simulink model "irep_force_control_m15"  (R2015a)
settings: Solver=ode3  StartTime=0.0  StopTime=inf  FixedStep=dt  RelTol=1e-3
InitFcn:
  | IREP_DEPENDENCY
  | init_omni
  | init_filters
  | init_invivo
  | init_telemanipulation
  | init_parker_xyz
  | init_magnetic_tracker
  | init_loadcell
  | init_scopes
  | init_homing
  | init_force_control
  | init_xpc_invivo_simu
undefined symbols (not defined in the file): ang_vel_scale, B_simu, beta, camera_home_voltage, counter_offset, dt, dt_trakstar, E_Y, encoder_counts, epsilon_robust_inverse, FS_LUT_TAU, FS_LUT_WE, gear_ratio, HomingFineEps, HomingRoughEps, HomingRoughVelocity, I1_primary, I1_secondary, I2_primary, I2_secondary, irep_parameters_left, irep_parameters_right, joystick_filter_coeffs, K_d, K_i, K_naive_inv, K_p, k_right, L1l, L1r, L2l, L2r, L_zeus, left_arm_home_voltage, left_x0_parallelogram, LeftArmHomingDirectionVector, LeftArmHomingIntGain, lin_vel_scale, LOADCELL_BIAS, LOADCELL_GAIN, max_conf_space_speed, N_joystick, N_pots, N_trakstar, OmegaMax, OmegaMin, orientation_epsilon, position_epsilon, pots_filter_coeffs, q_eps_backlash, quadrature_mode, r, right_arm_home_voltage, RightArmHomingDirectionVector, RightArmHomingIntGain, screw_pitch, statics_param, tau_compression_bias, tau_compression_gains, tau_neutral_deadband ... (+16)
libraries: slrtlib x39, simulink x23, xpcobsoletelib x23, xpcconteclib x23, xpcrtudplib x12, xpcmeasurementcomputinglib x6, dspswit3 x2, dspsigops x1
(part 5 of 7)

== system irep_force_control_m15/Trajectory Planner/Right Arm/High Level/Actuation Compensation/Grad U2 ==
  conf space : Inport
  q : Inport  Port=2
  Compute grad U : MATLAB Function  TreatAsAtomicUnit=on
  Constant : Constant  Value=L2r  SampleTime=dt
  E_Y : Constant  Value=E_Y  SampleTime=dt
  Ip : Constant  Value=I2_primary  SampleTime=dt
  Is : Constant  Value=I2_secondary  SampleTime=dt
  beta : Constant  Value=beta  SampleTime=dt
  r : Constant  Value=r  SampleTime=dt
  theta_0 : Constant  Value=theta0  SampleTime=dt
  grad_U : Outport
  wires:
  Is/1 -> Compute grad U/7(Is)
  q/1 -> Compute grad U/2(q)
  conf space/1 -> Compute grad U/1(conf_space)
  Compute grad U/1(grad_U) -> grad_U/1
  E_Y/1 -> Compute grad U/5(E_Y)
  Ip/1 -> Compute grad U/6(Ip)
  r/1 -> Compute grad U/4(r)
  theta_0/1 -> Compute grad U/8(theta_0)
  beta/1 -> Compute grad U/9(beta)
  Constant/1 -> Compute grad U/3(L_p)

== system irep_force_control_m15/Trajectory Planner/Right Arm/High Level/Actuation Compensation/Parallelogram Backlash Compensatior ==
  q des : Inport
  Backlash Compensator : MATLAB Function  TreatAsAtomicUnit=on
  Bus Selector : BusSelector  OutputSignals=q2;q3
  Discrete Derivative : simulink/Discrete/Discrete Derivative  gainval=1.0  ICPrevScaledInput=0.0  InputProcessing=Inherited  OutMin=[]  OutMax=[]  OutDataType=fixdt(1, 16)  OutScaling=2^-10  DoSatur=off
  comp close : Constant  Value=0
  comp close1 : Constant  Value=0.6
  comp open : Constant  Value=0
  comp open1 : Constant  Value=-1.2
  epsilon : Outport
  wires:
  q des/1 -> Bus Selector/1
  Bus Selector/1 -> Discrete Derivative/1, Backlash Compensator/1(q_curr)  "<q2;q3>"
  Discrete Derivative/1 -> Backlash Compensator/2(q_dot_curr)  "q dot curr"
  Backlash Compensator/1(epsilon) -> epsilon/1
  comp open/1 -> Backlash Compensator/3(q1_comp_open)
  comp close/1 -> Backlash Compensator/4(q1_comp_close)
  comp open1/1 -> Backlash Compensator/5(q2_comp_open)
  comp close1/1 -> Backlash Compensator/6(q2_comp_close)

== system irep_force_control_m15/Trajectory Planner/Right Arm/High Level/Actuation Compensation/get q_dot sign ==
  conf_space_dot : Inport
  conf_space : Inport  Port=2
  Dead Zone : DeadZone  LowerValue=-1e-3  UpperValue=1e-3  SaturateOnIntegerOverflow=on
  Unit Delay : UnitDelay  SampleTime=-1
  compute q_dot : MATLAB Function  TreatAsAtomicUnit=on
  hold q dot : MATLAB Function  TreatAsAtomicUnit=on
  q_dot : Outport
  wires:
  conf_space_dot/1 -> compute q_dot/2(conf_space_dot)
  conf_space/1 -> compute q_dot/1(conf_space)
  hold q dot/1(q_dot_sign_out) -> q_dot/1, Unit Delay/1
  Unit Delay/1 -> hold q dot/2(q_dot_sign_prev)
  compute q_dot/1(q_dot) -> Dead Zone/1
  Dead Zone/1 -> hold q dot/1(q_dot_sign_in)

== system irep_force_control_m15/Trajectory Planner/Right Arm/High Level/Actuation Compensation/q_eps 5th order poly ==
  q_eps_ref : Inport
  enable : Inport  Port=2
  Constant : Constant  Value=q_eps_backlash
  Digital Clock : DigitalClock  SampleTime=dt
  Embedded MATLAB Function : MATLAB Function  TreatAsAtomicUnit=on
  Terminator : Terminator
  Unit Delay : UnitDelay  SampleTime=dt
  Unit Delay1 : UnitDelay  SampleTime=dt
  Unit Delay2 : UnitDelay  InitialCondition=zeros(9,1)  SampleTime=dt
  tf : Constant  Value=5  SampleTime=dt
  q_eps_des : Outport
  wires:
  Embedded MATLAB Function/3(confn) -> Unit Delay/1
  Unit Delay/1 -> Embedded MATLAB Function/5(conf)
  Embedded MATLAB Function/4(t0n) -> Unit Delay1/1
  Embedded MATLAB Function/5(p0n) -> Unit Delay2/1
  Unit Delay2/1 -> Embedded MATLAB Function/7(p0)
  Unit Delay1/1 -> Embedded MATLAB Function/6(t0)
  Digital Clock/1 -> Embedded MATLAB Function/4(tc)
  q_eps_ref/1 -> Embedded MATLAB Function/1(p_des)
  Embedded MATLAB Function/1(p) -> q_eps_des/1
  tf/1 -> Embedded MATLAB Function/3(tf)
  enable/1 -> Embedded MATLAB Function/8(enable)
  Constant/1 -> Embedded MATLAB Function/2(p_curr)
  Embedded MATLAB Function/2(pdot) -> Terminator/1

== system irep_force_control_m15/Trajectory Planner/Right Arm/High Level/Configuration Space/Parallelogram ==
  Enable : EnablePort
  5th Order Polynomial : Subsystem
  b_des : Constant  Value=[x0_parallelogram z0_parallelogram]  SampleTime=dt
  b1 : Outport
  wires:
  b_des/1 -> 5th Order Polynomial/1(b des)
  5th Order Polynomial/1(b) -> b1/1

== system irep_force_control_m15/Trajectory Planner/Right Arm/High Level/Configuration Space/Stem ==
  Enable : EnablePort
  5th Order Polynomial : Subsystem
  Terminator : Terminator
  enable : Constant  Value=0  SampleTime=dt
  psi des : Constant  Value=[pi/2;0;pi/2;0;0]  SampleTime=dt
  psi0 : Constant  Value=[pi/2;0;pi/2;0;0]  SampleTime=dt
  psi dot : Outport  InitialOutput=zeros(5,1)
  wires:
  5th Order Polynomial/2(psi dot) -> psi dot/1
  psi des/1 -> 5th Order Polynomial/1(psi des)
  psi0/1 -> 5th Order Polynomial/2(psi0)
  enable/1 -> 5th Order Polynomial/3(enable)
  5th Order Polynomial/1(psi) -> Terminator/1

== system irep_force_control_m15/Trajectory Planner/Right Arm/High Level/Inverse Istantaneous Kinematics/Coordination Module ==
  b1 : Inport
  q par : Inport  Port=2
  5-Bar Inverse Kinematics : MATLAB Function  TreatAsAtomicUnit=on
  Add : Sum  Inputs=+-  SampleTime=dt
  Coordination Block : MATLAB Function  TreatAsAtomicUnit=on
  L0 : Constant  Value=L_zeus  SampleTime=dt
  b0 : Constant  Value=[x0_parallelogram z0_parallelogram]  SampleTime=dt
  q1 : Outport
  "q2, q3" : Outport  Port=2
  wires:
  Add/1 -> "q2, q3"/1
  q par/1 -> Coordination Block/2(q_par)
  b1/1 -> Coordination Block/1(b1)
  Coordination Block/1(q1) -> q1/1
  5-Bar Inverse Kinematics/1(q) -> Add/2
  L0/1 -> Coordination Block/3(L0)
  b0/1 -> 5-Bar Inverse Kinematics/1(b1)
  Coordination Block/2(q23) -> Add/1

== system irep_force_control_m15/Trajectory Planner/Right Arm/High Level/Inverse Istantaneous Kinematics/Jaw Open//Close Module ==
  sensors : Inport
  Enable : EnablePort
  Bus Selector : BusSelector  OutputSignals=MSG_Type,gripper
  Jaw Open/Close : MATLAB Function  TreatAsAtomicUnit=on
  MTM_GP_max : Constant  Value=1.05
  MTM_GP_min : Constant  Value=-0.48
  Unit Delay : UnitDelay  SampleTime=-1
  Unit Delay1 : UnitDelay  SampleTime=-1
  q9 : Outport
  wires:
  sensors/1 -> Bus Selector/1
  Jaw Open/Close/1(y) -> Unit Delay/1, Unit Delay1/1
  Bus Selector/2 -> Jaw Open/Close/2(u)  "<gripper>"
  MTM_GP_max/1 -> Jaw Open/Close/3(MTM_GP_max)
  MTM_GP_min/1 -> Jaw Open/Close/4(MTM_GP_min)
  Bus Selector/1 -> Jaw Open/Close/1(MSG_valid)  "<MSG_Type>"
  Unit Delay/1 -> Jaw Open/Close/5(q9_prev)
  Unit Delay1/1 -> q9/1

== system irep_force_control_m15/Trajectory Planner/Right Arm/High Level/Task Space/Compute Weigths ==
  sensors : Inport
  conf space : Inport  Port=2
  Bus Selector : BusSelector  OutputSignals=b1 curr,psi curr
  Bus Selector1 : BusSelector  OutputSignals=foot switches
  joint limits : Constant  Value=[x0_parallelogram x0_parallelogram_max z0_parallelogram z0_parallelogram_max theta_min1 theta_max theta_min2 theta_max wrist_min wrist_max]  SampleTime=dt
  select weights : MATLAB Function  TreatAsAtomicUnit=on
  w_min : Constant  Value=w_min  SampleTime=dt
  weights : Outport
  wires:
  joint limits/1 -> select weights/3(joint_limits)
  Bus Selector/1 -> select weights/1(b1)  "<b1 curr>"
  Bus Selector/2 -> select weights/2(psi)  "<psi curr>"
  conf space/1 -> Bus Selector/1
  select weights/1(W) -> weights/1
  w_min/1 -> select weights/4(w_min)
  sensors/1 -> Bus Selector1/1
  Bus Selector1/1 -> select weights/5(foot_switches)  "<foot switches>"

== system irep_force_control_m15/Trajectory Planner/Right Arm/High Level/Task Space/Desired Twist Module ==
  note: Desired Twist Module v 1.1 - © 2011 Andrea Bajo, Nabil Simaan
  current pose : Inport
  des pose : Inport  Port=2
  Bus Selector1 : BusSelector  OutputSignals=p in world,R in world
  Bus Selector2 : BusSelector  OutputSignals=position,R,MSG_Type
  Compute Twist : MATLAB Function  TreatAsAtomicUnit=on
  Omega Max : Constant  Value=OmegaMax  SampleTime=dt
  Omega Min : Constant  Value=OmegaMin  SampleTime=dt
  V Max : Constant  Value=Vmax  SampleTime=dt
  V Min : Constant  Value=Vmin  SampleTime=dt
  ang vel scale : Constant  Value=ang_vel_scale  SampleTime=dt
  lin vel scale : Constant  Value=lin_vel_scale  SampleTime=dt
  orientation epsilon : Constant  Value=orientation_epsilon  SampleTime=dt
  position epsilon : Constant  Value=position_epsilon  SampleTime=dt
  x des : Outport
  wires:
  Bus Selector1/1 -> Compute Twist/4(p_curr)  "<p in world>"
  Compute Twist/1(x_des) -> x des/1
  current pose/1 -> Bus Selector1/1
  Bus Selector1/2 -> Compute Twist/5(R_curr)  "<R in world>"
  Bus Selector2/1 -> Compute Twist/1(p_des)  "<position>"
  Bus Selector2/2 -> Compute Twist/2(R_des)  "<R>"
  des pose/1 -> Bus Selector2/1
  Bus Selector2/3 -> Compute Twist/3(MSG_Type)  "<MSG_Type>"
  V Max/1 -> Compute Twist/6(Vmax)
  Omega Max/1 -> Compute Twist/10(OmegaMax)
  V Min/1 -> Compute Twist/7(Vmin)
  Omega Min/1 -> Compute Twist/11(OmegaMin)
  position epsilon/1 -> Compute Twist/8(position_epsilon)
  orientation epsilon/1 -> Compute Twist/12(orientation_epsilon)
  lin vel scale/1 -> Compute Twist/9(lin_vel_scale)
  ang vel scale/1 -> Compute Twist/13(ang_vel_scale)

== system irep_force_control_m15/Trajectory Planner/Right Arm/High Level/Task Space/Direct Kinematics IREP ==
  "b1, psi" : Inport
  Bus Creator : BusCreator  Inputs=2
  Bus Selector : BusSelector  OutputSignals=Parker insertion stage,b1 curr,psi curr
  Direct Kinematic IREP : MATLAB Function  TreatAsAtomicUnit=on
  IREP parameters : Constant  Value=irep_parameters_right  SampleTime=dt
  Current Pose : Outport
  wires:
  "b1, psi"/1 -> Bus Selector/1
  Bus Selector/2 -> Direct Kinematic IREP/2(b1)  "<b1 curr>"
  Bus Selector/3 -> Direct Kinematic IREP/3(psi)  "<psi curr>"
  Direct Kinematic IREP/1(p) -> Bus Creator/1  "p in world"
  Direct Kinematic IREP/2(R) -> Bus Creator/2  "R in world"
  Bus Creator/1 -> Current Pose/1
  IREP parameters/1 -> Direct Kinematic IREP/4(parameters)
  Bus Selector/1 -> Direct Kinematic IREP/1(b0)  "<Parker insertion stage>"

== system irep_force_control_m15/Trajectory Planner/Right Arm/High Level/Task Space/Jxpsi Inverse IREP ==
  x des : Inport
  weights : Inport  Port=2
  "b1, psi" : Inport  Port=3
  Bus Selector : BusSelector  OutputSignals=Parker insertion stage,b1 curr,psi curr
  IREP parameters : Constant  Value=irep_parameters_right  SampleTime=dt
  Jxpsi Inverse IREP : MATLAB Function  TreatAsAtomicUnit=on
  epsilon : Constant  Value=epsilon_robust_inverse  SampleTime=dt
  max conf space speed : Constant  Value=max_conf_space_speed  SampleTime=dt
  conf dot des : Outport  PortDimensions=[8 1]
  wires:
  IREP parameters/1 -> Jxpsi Inverse IREP/5(parameters)
  x des/1 -> Jxpsi Inverse IREP/1(x_des)
  Bus Selector/3 -> Jxpsi Inverse IREP/4(psi)  "<psi curr>"
  Bus Selector/2 -> Jxpsi Inverse IREP/3(b1)  "<b1 curr>"
  "b1, psi"/1 -> Bus Selector/1
  Jxpsi Inverse IREP/1(conf_space_dot) -> conf dot des/1
  epsilon/1 -> Jxpsi Inverse IREP/7(epsilon_in)
  weights/1 -> Jxpsi Inverse IREP/6(weights)
  Bus Selector/1 -> Jxpsi Inverse IREP/2(b0)  "<Parker insertion stage>"
  max conf space speed/1 -> Jxpsi Inverse IREP/8(max_ang_speed)

== system irep_force_control_m15/Trajectory Planner/Right Arm/High Level/Task Space/Receive Desired Pose from MTM ==
  note: Telemanipulation Module v 1.0 - © COPYRIGHT 2010 Andrea Bajo, Nabil Simaan
  Master : Inport
  Bus Creator : BusCreator
  Bus Selector : BusSelector  OutputSignals=position,orientation (quat),MSG_Type,gripper
  Quaternion To Rotation : MATLAB Function  TreatAsAtomicUnit=on
  "pose, flags" : Outport
  wires:
  Bus Creator/1 -> "pose, flags"/1
  Master/1 -> Bus Selector/1
  Bus Selector/1 -> Bus Creator/1  "<position>"
  Quaternion To Rotation/1(R) -> Bus Creator/2
  Bus Selector/2 -> Quaternion To Rotation/1(quat)  "<orientation (quat)>"
  Bus Selector/3 -> Bus Creator/3  "<MSG_Type>"
  Bus Selector/4 -> Bus Creator/4  "<gripper>"

== system irep_force_control_m15/Trajectory Planner/Right Arm/High Level/Task Space/right task space scope ==
  des : Inport
  Bus Selector7 : BusSelector  OutputSignals=position,R,gripper,MSG_Type
  Gain : Gain
  Mux : Mux  Inputs=5
  R_to_axis_angle1 : MATLAB Function  TreatAsAtomicUnit=on
  right task space : slrtlib/Displays and Logging/Scope   scopeno=26  scopetype=Host  autostart=on  viewmode=Numerical  formatstr=scope_format_right_task_space_des  grid=on  ylimits=[0,0]  nosamples=10  noprepostsamples=0  interleave=1  triggermode=FreeRun  triggersignal=1  trigsignalfromport=off  triggerlevel=0.0  triggerslope=Either  triggerscope=1  triggersample=0  filename=weights1.dat  mode=Lazy  writesize=512  autorestart=off  dynamicfilemode=off  maxwritefilesize=512*1024^2
  wires:
  Mux/1 -> Gain/1
  des/1 -> Bus Selector7/1
  Bus Selector7/2 -> R_to_axis_angle1/1(R)  "<R>"
  Gain/1 -> right task space/1
  Bus Selector7/3 -> Mux/4  "<gripper>"
  R_to_axis_angle1/1(n_vec) -> Mux/2
  R_to_axis_angle1/2(theta) -> Mux/3
  Bus Selector7/1 -> Mux/1  "<position>"
  Bus Selector7/4 -> Mux/5  "<MSG_Type>"

== system irep_force_control_m15/Trajectory Planner/Right Arm/Low Level/Home Procedure/Fine Homing - Integral Control ==
  error : Inport
  Enable : EnablePort  StatesWhenEnabling=reset
  Discrete-Time Integrator : DiscreteIntegrator  SampleTime=dt  LimitOutput=on  UpperSaturationLimit=8  LowerSaturationLimit=-8
  Integral Gain : Gain  Gain=diag(RightArmHomingIntGain)  Multiplication=Matrix(K*u)  SampleTime=dt
  q_des_fine : Outport  InitialOutput=zeros(9,1)
  wires:
  error/1 -> Integral Gain/1
  Discrete-Time Integrator/1 -> q_des_fine/1
  Integral Gain/1 -> Discrete-Time Integrator/1

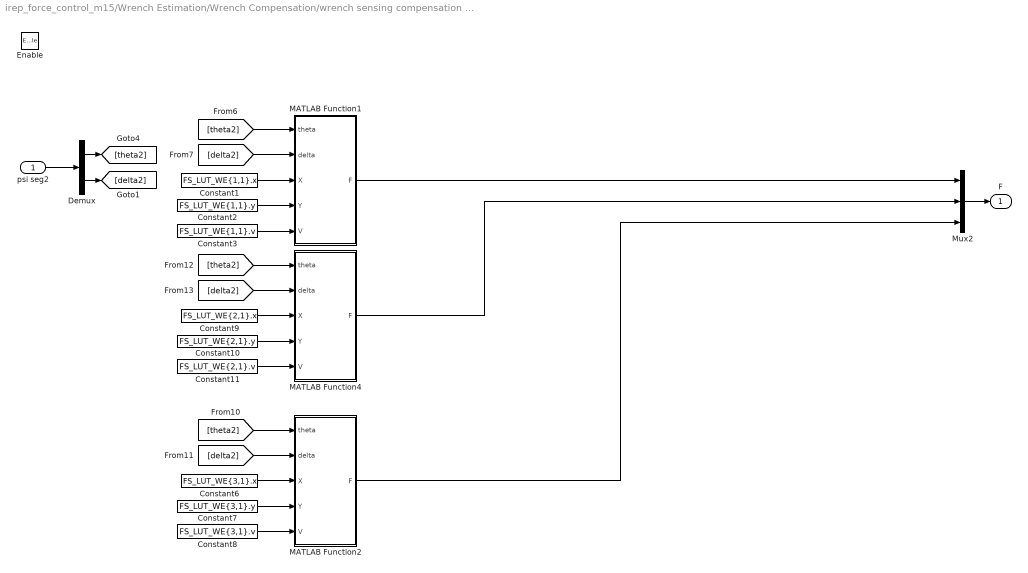
== system irep_force_control_m15/Wrench Estimation/Wrench Compensation/wrench sensing compensation LUT/wrench seg2 bias LUT/Interp2 Case A ==
  psi seg2 : Inport
  Enable : EnablePort
  Constant1 : Constant  Value=FS_LUT_WE{1,1}.x  VectorParams1D=off
  Constant10 : Constant  Value=FS_LUT_WE{2,1}.y  VectorParams1D=off
  Constant11 : Constant  Value=FS_LUT_WE{2,1}.v  VectorParams1D=off
  Constant2 : Constant  Value=FS_LUT_WE{1,1}.y  VectorParams1D=off
  Constant3 : Constant  Value=FS_LUT_WE{1,1}.v  VectorParams1D=off
  Constant6 : Constant  Value=FS_LUT_WE{3,1}.x  VectorParams1D=off
  Constant7 : Constant  Value=FS_LUT_WE{3,1}.y  VectorParams1D=off
  Constant8 : Constant  Value=FS_LUT_WE{3,1}.v  VectorParams1D=off
  Constant9 : Constant  Value=FS_LUT_WE{2,1}.x  VectorParams1D=off
  Demux : Demux  Outputs=2
  MATLAB Function1 : MATLAB Function  TreatAsAtomicUnit=on
  MATLAB Function2 : MATLAB Function  TreatAsAtomicUnit=on
  MATLAB Function4 : MATLAB Function  TreatAsAtomicUnit=on
  Mux2 : Mux  Inputs=3
  F : Outport
  wires:
  Constant3/1 -> MATLAB Function1/5(V)
  Constant2/1 -> MATLAB Function1/4(Y)
  Constant1/1 -> MATLAB Function1/3(X)
  [delta2] -> MATLAB Function1/2(delta)
  [theta2] -> MATLAB Function1/1(theta)
  Constant11/1 -> MATLAB Function4/5(V)
  Constant10/1 -> MATLAB Function4/4(Y)
  Constant9/1 -> MATLAB Function4/3(X)
  [delta2] -> MATLAB Function4/2(delta)
  [theta2] -> MATLAB Function4/1(theta)
  Constant8/1 -> MATLAB Function2/5(V)
  Constant7/1 -> MATLAB Function2/4(Y)
  Constant6/1 -> MATLAB Function2/3(X)
  [delta2] -> MATLAB Function2/2(delta)
  [theta2] -> MATLAB Function2/1(theta)
  MATLAB Function4/1(F) -> Mux2/2
  Mux2/1 -> F/1
  MATLAB Function1/1(F) -> Mux2/1
  MATLAB Function2/1(F) -> Mux2/3
  Demux/2 -> [delta2]
  Demux/1 -> [theta2]
  psi seg2/1 -> Demux/1

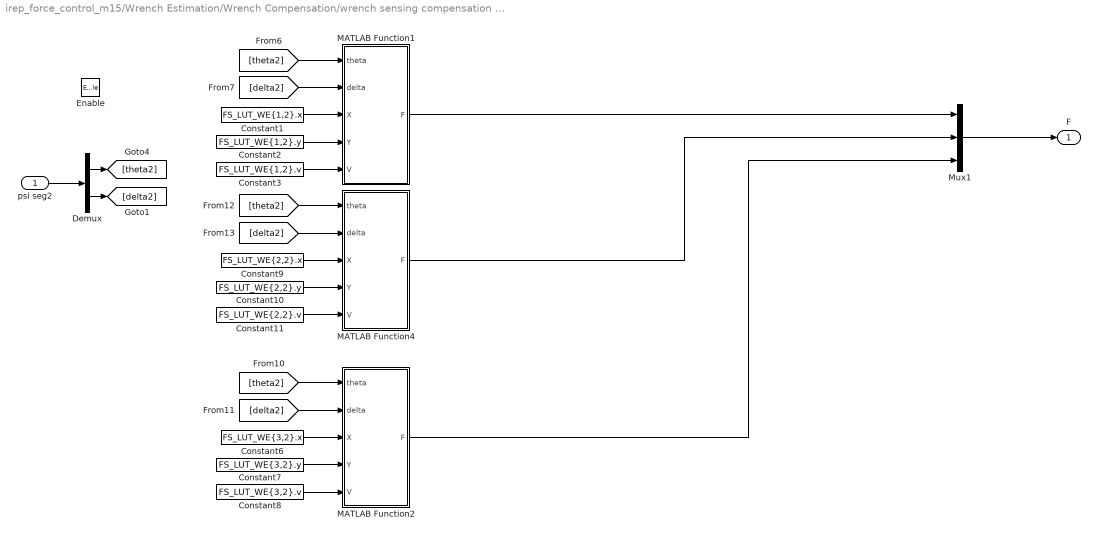
== system irep_force_control_m15/Wrench Estimation/Wrench Compensation/wrench sensing compensation LUT/wrench seg2 bias LUT/Interp2 Case B ==
  psi seg2 : Inport
  Enable : EnablePort
  Constant1 : Constant  Value=FS_LUT_WE{1,2}.x  VectorParams1D=off
  Constant10 : Constant  Value=FS_LUT_WE{2,2}.y  VectorParams1D=off
  Constant11 : Constant  Value=FS_LUT_WE{2,2}.v  VectorParams1D=off
  Constant2 : Constant  Value=FS_LUT_WE{1,2}.y  VectorParams1D=off
  Constant3 : Constant  Value=FS_LUT_WE{1,2}.v  VectorParams1D=off
  Constant6 : Constant  Value=FS_LUT_WE{3,2}.x  VectorParams1D=off
  Constant7 : Constant  Value=FS_LUT_WE{3,2}.y  VectorParams1D=off
  Constant8 : Constant  Value=FS_LUT_WE{3,2}.v  VectorParams1D=off
  Constant9 : Constant  Value=FS_LUT_WE{2,2}.x  VectorParams1D=off
  Demux : Demux  Outputs=2
  MATLAB Function1 : MATLAB Function  TreatAsAtomicUnit=on
  MATLAB Function2 : MATLAB Function  TreatAsAtomicUnit=on
  MATLAB Function4 : MATLAB Function  TreatAsAtomicUnit=on
  Mux1 : Mux  Inputs=3
  F : Outport
  wires:
  Constant3/1 -> MATLAB Function1/5(V)
  Constant2/1 -> MATLAB Function1/4(Y)
  Constant1/1 -> MATLAB Function1/3(X)
  [delta2] -> MATLAB Function1/2(delta)
  [theta2] -> MATLAB Function1/1(theta)
  Constant11/1 -> MATLAB Function4/5(V)
  Constant10/1 -> MATLAB Function4/4(Y)
  Constant9/1 -> MATLAB Function4/3(X)
  [delta2] -> MATLAB Function4/2(delta)
  [theta2] -> MATLAB Function4/1(theta)
  Constant8/1 -> MATLAB Function2/5(V)
  Constant7/1 -> MATLAB Function2/4(Y)
  Constant6/1 -> MATLAB Function2/3(X)
  [delta2] -> MATLAB Function2/2(delta)
  [theta2] -> MATLAB Function2/1(theta)
  MATLAB Function4/1(F) -> Mux1/2
  Mux1/1 -> F/1
  MATLAB Function1/1(F) -> Mux1/1
  MATLAB Function2/1(F) -> Mux1/3
  Demux/2 -> [delta2]
  Demux/1 -> [theta2]
  psi seg2/1 -> Demux/1

== system irep_force_control_m15/Wrench Estimation/Wrench Compensation/wrench sensing compensation LUT/wrench seg2 bias LUT/Interp2 Case C ==
  psi seg2 : Inport
  Enable : EnablePort
  Constant1 : Constant  Value=FS_LUT_WE{1,3}.x  VectorParams1D=off
  Constant10 : Constant  Value=FS_LUT_WE{2,3}.y  VectorParams1D=off
  Constant11 : Constant  Value=FS_LUT_WE{2,3}.v  VectorParams1D=off
  Constant2 : Constant  Value=FS_LUT_WE{1,3}.y  VectorParams1D=off
  Constant3 : Constant  Value=FS_LUT_WE{1,3}.v  VectorParams1D=off
  Constant6 : Constant  Value=FS_LUT_WE{3,3}.x  VectorParams1D=off
  Constant7 : Constant  Value=FS_LUT_WE{3,3}.y  VectorParams1D=off
  Constant8 : Constant  Value=FS_LUT_WE{3,3}.v  VectorParams1D=off
  Constant9 : Constant  Value=FS_LUT_WE{2,3}.x  VectorParams1D=off
  Demux : Demux  Outputs=2
  MATLAB Function1 : MATLAB Function  TreatAsAtomicUnit=on
  MATLAB Function2 : MATLAB Function  TreatAsAtomicUnit=on
  MATLAB Function4 : MATLAB Function  TreatAsAtomicUnit=on
  Mux2 : Mux  Inputs=3
  F1 : Outport
  wires:
  Constant3/1 -> MATLAB Function1/5(V)
  Constant2/1 -> MATLAB Function1/4(Y)
  Constant1/1 -> MATLAB Function1/3(X)
  [delta2] -> MATLAB Function1/2(delta)
  [theta2] -> MATLAB Function1/1(theta)
  Constant11/1 -> MATLAB Function4/5(V)
  Constant10/1 -> MATLAB Function4/4(Y)
  Constant9/1 -> MATLAB Function4/3(X)
  [delta2] -> MATLAB Function4/2(delta)
  [theta2] -> MATLAB Function4/1(theta)
  Constant8/1 -> MATLAB Function2/5(V)
  Constant7/1 -> MATLAB Function2/4(Y)
  Constant6/1 -> MATLAB Function2/3(X)
  [delta2] -> MATLAB Function2/2(delta)
  [theta2] -> MATLAB Function2/1(theta)
  MATLAB Function4/1(F) -> Mux2/2
  Mux2/1 -> F1/1
  MATLAB Function1/1(F) -> Mux2/1
  MATLAB Function2/1(F) -> Mux2/3
  Demux/2 -> [delta2]
  Demux/1 -> [theta2]
  psi seg2/1 -> Demux/1

== system irep_force_control_m15/Wrench Estimation/Wrench Compensation/wrench sensing compensation LUT/wrench seg2 bias LUT/Interp2 Case D ==
  psi seg2 : Inport
  Enable : EnablePort
  Constant1 : Constant  Value=FS_LUT_WE{1,4}.x  VectorParams1D=off
  Constant10 : Constant  Value=FS_LUT_WE{2,4}.y  VectorParams1D=off
  Constant11 : Constant  Value=FS_LUT_WE{2,4}.v  VectorParams1D=off
  Constant2 : Constant  Value=FS_LUT_WE{1,4}.y  VectorParams1D=off
  Constant3 : Constant  Value=FS_LUT_WE{1,4}.v  VectorParams1D=off
  Constant6 : Constant  Value=FS_LUT_WE{3,4}.x  VectorParams1D=off
  Constant7 : Constant  Value=FS_LUT_WE{3,4}.y  VectorParams1D=off
  Constant8 : Constant  Value=FS_LUT_WE{3,4}.v  VectorParams1D=off
  Constant9 : Constant  Value=FS_LUT_WE{2,4}.x  VectorParams1D=off
  Demux : Demux  Outputs=2
  MATLAB Function1 : MATLAB Function  TreatAsAtomicUnit=on
  MATLAB Function2 : MATLAB Function  TreatAsAtomicUnit=on
  MATLAB Function4 : MATLAB Function  TreatAsAtomicUnit=on
  Mux2 : Mux  Inputs=3
  F1 : Outport
  wires:
  Constant3/1 -> MATLAB Function1/5(V)
  Constant2/1 -> MATLAB Function1/4(Y)
  Constant1/1 -> MATLAB Function1/3(X)
  [delta2] -> MATLAB Function1/2(delta)
  [theta2] -> MATLAB Function1/1(theta)
  Constant11/1 -> MATLAB Function4/5(V)
  Constant10/1 -> MATLAB Function4/4(Y)
  Constant9/1 -> MATLAB Function4/3(X)
  [delta2] -> MATLAB Function4/2(delta)
  [theta2] -> MATLAB Function4/1(theta)
  Constant8/1 -> MATLAB Function2/5(V)
  Constant7/1 -> MATLAB Function2/4(Y)
  Constant6/1 -> MATLAB Function2/3(X)
  [delta2] -> MATLAB Function2/2(delta)
  [theta2] -> MATLAB Function2/1(theta)
  MATLAB Function4/1(F) -> Mux2/2
  Mux2/1 -> F1/1
  MATLAB Function1/1(F) -> Mux2/1
  MATLAB Function2/1(F) -> Mux2/3
  Demux/2 -> [delta2]
  Demux/1 -> [theta2]
  psi seg2/1 -> Demux/1

== system irep_force_control_m15/Wrench Estimation/Wrench Compensation/wrench sensing compensation LUT/wrench seg2 bias LUT/LUT Case A ==
  psi seg2 : Inport
  Enable : EnablePort
  Demux : Demux  Outputs=2
  Mux1 : Mux  Inputs=3
  XA_Lookup : Lookup_n-D  BreakpointsForDimension1=FS_LUT_WE{1,1}.x  BreakpointsForDimension2=FS_LUT_WE{1,1}.y  Table=FS_LUT_WE{1,1}.v  InternalRulePriority=Speed  RndMeth=Simplest  InputSameDT=on
  YA_Lookup : Lookup_n-D  BreakpointsForDimension1=FS_LUT_WE{2,1}.x  BreakpointsForDimension2=FS_LUT_WE{2,1}.y  Table=FS_LUT_WE{2,1}.v  InternalRulePriority=Speed  RndMeth=Simplest  InputSameDT=on
  ZA_Lookup : Lookup_n-D  BreakpointsForDimension1=FS_LUT_WE{3,1}.x  BreakpointsForDimension2=FS_LUT_WE{3,1}.y  Table=FS_LUT_WE{3,1}.v  InternalRulePriority=Speed  RndMeth=Simplest  InputSameDT=on
  F : Outport
  wires:
  YA_Lookup/1 -> Mux1/2
  [theta2] -> XA_Lookup/1
  [delta2] -> XA_Lookup/2
  [theta2] -> YA_Lookup/1
  [delta2] -> ZA_Lookup/2
  [delta2] -> YA_Lookup/2
  ZA_Lookup/1 -> Mux1/3
  [theta2] -> ZA_Lookup/1
  XA_Lookup/1 -> Mux1/1
  psi seg2/1 -> Demux/1
  Demux/1 -> [theta2]
  Demux/2 -> [delta2]
  Mux1/1 -> F/1
  ? -> ?

== system irep_force_control_m15/Wrench Estimation/Wrench Compensation/wrench sensing compensation LUT/wrench seg2 bias LUT/LUT Case B ==
  psi seg2 : Inport
  Enable : EnablePort
  Demux : Demux  Outputs=2
  Mux2 : Mux  Inputs=3
  XA_Lookup : Lookup_n-D  BreakpointsForDimension1=FS_LUT_WE{1,2}.x  BreakpointsForDimension2=FS_LUT_WE{1,2}.y  Table=FS_LUT_WE{1,2}.v  InternalRulePriority=Speed  RndMeth=Simplest  InputSameDT=on
  YA_Lookup : Lookup_n-D  BreakpointsForDimension1=FS_LUT_WE{2,2}.x  BreakpointsForDimension2=FS_LUT_WE{2,2}.y  Table=FS_LUT_WE{2,2}.v  InternalRulePriority=Speed  RndMeth=Simplest  InputSameDT=on
  ZA_Lookup : Lookup_n-D  BreakpointsForDimension1=FS_LUT_WE{3,2}.x  BreakpointsForDimension2=FS_LUT_WE{3,2}.y  Table=FS_LUT_WE{3,2}.v  InternalRulePriority=Speed  RndMeth=Simplest  InputSameDT=on
  F : Outport
  wires:
  YA_Lookup/1 -> Mux2/2
  [theta2] -> XA_Lookup/1
  [delta2] -> XA_Lookup/2
  [theta2] -> YA_Lookup/1
  [delta2] -> ZA_Lookup/2
  [delta2] -> YA_Lookup/2
  ZA_Lookup/1 -> Mux2/3
  [theta2] -> ZA_Lookup/1
  XA_Lookup/1 -> Mux2/1
  psi seg2/1 -> Demux/1
  Demux/1 -> [theta2]
  Demux/2 -> [delta2]
  Mux2/1 -> F/1

== system irep_force_control_m15/Wrench Estimation/Wrench Compensation/wrench sensing compensation LUT/wrench seg2 bias LUT/LUT Case C ==
  psi seg2 : Inport
  Enable : EnablePort
  Demux : Demux  Outputs=2
  Mux3 : Mux  Inputs=3
  XA_Lookup : Lookup_n-D  BreakpointsForDimension1=FS_LUT_WE{1,3}.x  BreakpointsForDimension2=FS_LUT_WE{1,3}.y  Table=FS_LUT_WE{1,3}.v  InternalRulePriority=Speed  RndMeth=Simplest  InputSameDT=on
  YA_Lookup : Lookup_n-D  BreakpointsForDimension1=FS_LUT_WE{2,3}.x  BreakpointsForDimension2=FS_LUT_WE{2,3}.y  Table=FS_LUT_WE{2,3}.v  InternalRulePriority=Speed  RndMeth=Simplest  InputSameDT=on
  ZA_Lookup : Lookup_n-D  BreakpointsForDimension1=FS_LUT_WE{3,3}.x  BreakpointsForDimension2=FS_LUT_WE{3,3}.y  Table=FS_LUT_WE{3,3}.v  InternalRulePriority=Speed  RndMeth=Simplest  InputSameDT=on
  F : Outport
  wires:
  YA_Lookup/1 -> Mux3/2
  [theta2] -> XA_Lookup/1
  [delta2] -> XA_Lookup/2
  [theta2] -> YA_Lookup/1
  [delta2] -> ZA_Lookup/2
  [delta2] -> YA_Lookup/2
  ZA_Lookup/1 -> Mux3/3
  [theta2] -> ZA_Lookup/1
  XA_Lookup/1 -> Mux3/1
  psi seg2/1 -> Demux/1
  Demux/1 -> [theta2]
  Demux/2 -> [delta2]
  Mux3/1 -> F/1

== system irep_force_control_m15/Wrench Estimation/Wrench Compensation/wrench sensing compensation LUT/wrench seg2 bias LUT/LUT Case D ==
  psi seg2 : Inport
  Enable : EnablePort
  Demux : Demux  Outputs=2
  Mux4 : Mux  Inputs=3
  XA_Lookup : Lookup_n-D  BreakpointsForDimension1=FS_LUT_WE{1,4}.x  BreakpointsForDimension2=FS_LUT_WE{1,4}.y  Table=FS_LUT_WE{1,4}.v  InternalRulePriority=Speed  RndMeth=Simplest  InputSameDT=on
  YA_Lookup : Lookup_n-D  BreakpointsForDimension1=FS_LUT_WE{2,4}.x  BreakpointsForDimension2=FS_LUT_WE{2,4}.y  Table=FS_LUT_WE{2,4}.v  InternalRulePriority=Speed  RndMeth=Simplest  InputSameDT=on
  ZA_Lookup : Lookup_n-D  BreakpointsForDimension1=FS_LUT_WE{3,4}.x  BreakpointsForDimension2=FS_LUT_WE{3,4}.y  Table=FS_LUT_WE{3,4}.v  InternalRulePriority=Speed  RndMeth=Simplest  InputSameDT=on
  F : Outport
  wires:
  YA_Lookup/1 -> Mux4/2
  [theta2] -> XA_Lookup/1
  [delta2] -> XA_Lookup/2
  [theta2] -> YA_Lookup/1
  [delta2] -> ZA_Lookup/2
  [delta2] -> YA_Lookup/2
  ZA_Lookup/1 -> Mux4/3
  [theta2] -> ZA_Lookup/1
  XA_Lookup/1 -> Mux4/1
  psi seg2/1 -> Demux/1
  Demux/1 -> [theta2]
  Demux/2 -> [delta2]
  Mux4/1 -> F/1

== system irep_force_control_m15/Wrench Estimation/tau sensing compensation/tau sensing compensation LUT/tau seg2 bias LUT/tau5_bias_neg ==
  psi seg2 : Inport
  Enable : EnablePort
  Constant1 : Constant  Value=FS_LUT_TAU{5,2}.x  VectorParams1D=off
  Constant2 : Constant  Value=FS_LUT_TAU{5,2}.y  VectorParams1D=off
  Constant3 : Constant  Value=FS_LUT_TAU{5,2}.v  VectorParams1D=off
  Demux : Demux  Outputs=2
  MATLAB Function1 : MATLAB Function  TreatAsAtomicUnit=on
  Tau_Bias : Outport
  wires:
  Demux/2 -> [delta2]
  Demux/1 -> [theta2]
  psi seg2/1 -> Demux/1
  MATLAB Function1/1(F) -> Tau_Bias/1
  [delta2] -> MATLAB Function1/2(delta)
  [theta2] -> MATLAB Function1/1(theta)
  Constant2/1 -> MATLAB Function1/4(Y)
  Constant3/1 -> MATLAB Function1/5(V)
  Constant1/1 -> MATLAB Function1/3(X)

== system irep_force_control_m15/Wrench Estimation/tau sensing compensation/tau sensing compensation LUT/tau seg2 bias LUT/tau5_bias_pos ==
  psi seg2 : Inport
  Enable : EnablePort
  Constant4 : Constant  Value=FS_LUT_TAU{5,1}.x  VectorParams1D=off
  Constant5 : Constant  Value=FS_LUT_TAU{5,1}.y  VectorParams1D=off
  Constant6 : Constant  Value=FS_LUT_TAU{5,1}.v  VectorParams1D=off
  Demux : Demux  Outputs=2
  MATLAB Function2 : MATLAB Function  TreatAsAtomicUnit=on
  Tau_Bias : Outport
  wires:
  Demux/2 -> [delta2]
  Demux/1 -> [theta2]
  psi seg2/1 -> Demux/1
  Constant6/1 -> MATLAB Function2/5(V)
  MATLAB Function2/1(F) -> Tau_Bias/1
  [delta2] -> MATLAB Function2/2(delta)
  [theta2] -> MATLAB Function2/1(theta)
  Constant4/1 -> MATLAB Function2/3(X)
  Constant5/1 -> MATLAB Function2/4(Y)

== system irep_force_control_m15/Wrench Estimation/tau sensing compensation/tau sensing compensation LUT/tau seg2 bias LUT/tau6_bias_neg ==
  psi seg2 : Inport
  Enable : EnablePort
  Constant1 : Constant  Value=FS_LUT_TAU{6,2}.x  VectorParams1D=off
  Constant2 : Constant  Value=FS_LUT_TAU{6,2}.y  VectorParams1D=off
  Constant3 : Constant  Value=FS_LUT_TAU{6,2}.v  VectorParams1D=off
  Demux : Demux  Outputs=2
  MATLAB Function1 : MATLAB Function  TreatAsAtomicUnit=on
  Tau_Bias : Outport
  wires:
  Demux/2 -> [delta2]
  Demux/1 -> [theta2]
  psi seg2/1 -> Demux/1
  Constant1/1 -> MATLAB Function1/3(X)
  Constant3/1 -> MATLAB Function1/5(V)
  Constant2/1 -> MATLAB Function1/4(Y)
  [theta2] -> MATLAB Function1/1(theta)
  [delta2] -> MATLAB Function1/2(delta)
  MATLAB Function1/1(F) -> Tau_Bias/1

== system irep_force_control_m15/Wrench Estimation/tau sensing compensation/tau sensing compensation LUT/tau seg2 bias LUT/tau6_bias_pos ==
  psi seg2 : Inport
  Enable : EnablePort
  Constant4 : Constant  Value=FS_LUT_TAU{6,1}.x  VectorParams1D=off
  Constant5 : Constant  Value=FS_LUT_TAU{6,1}.y  VectorParams1D=off
  Constant6 : Constant  Value=FS_LUT_TAU{6,1}.v  VectorParams1D=off
  Demux : Demux  Outputs=2
  MATLAB Function2 : MATLAB Function  TreatAsAtomicUnit=on
  Tau_Bias : Outport
  wires:
  Demux/2 -> [delta2]
  Demux/1 -> [theta2]
  psi seg2/1 -> Demux/1
  Constant5/1 -> MATLAB Function2/4(Y)
  Constant4/1 -> MATLAB Function2/3(X)
  [theta2] -> MATLAB Function2/1(theta)
  [delta2] -> MATLAB Function2/2(delta)
  MATLAB Function2/1(F) -> Tau_Bias/1
  Constant6/1 -> MATLAB Function2/5(V)

== system irep_force_control_m15/Wrench Estimation/tau sensing compensation/tau sensing compensation LUT/tau seg2 bias LUT/tau7_bias_neg ==
  psi seg2 : Inport
  Enable : EnablePort
  Constant1 : Constant  Value=FS_LUT_TAU{7,2}.x  VectorParams1D=off
  Constant2 : Constant  Value=FS_LUT_TAU{7,2}.y  VectorParams1D=off
  Constant3 : Constant  Value=FS_LUT_TAU{7,2}.v  VectorParams1D=off
  Demux : Demux  Outputs=2
  MATLAB Function1 : MATLAB Function  TreatAsAtomicUnit=on
  Tau_Bias : Outport
  wires:
  Constant1/1 -> MATLAB Function1/3(X)
  Constant3/1 -> MATLAB Function1/5(V)
  Constant2/1 -> MATLAB Function1/4(Y)
  [theta2] -> MATLAB Function1/1(theta)
  [delta2] -> MATLAB Function1/2(delta)
  MATLAB Function1/1(F) -> Tau_Bias/1
  psi seg2/1 -> Demux/1
  Demux/1 -> [theta2]
  Demux/2 -> [delta2]

== system irep_force_control_m15/Wrench Estimation/tau sensing compensation/tau sensing compensation LUT/tau seg2 bias LUT/tau7_bias_pos ==
  psi seg2 : Inport
  Enable : EnablePort
  Constant4 : Constant  Value=FS_LUT_TAU{7,1}.x  VectorParams1D=off
  Constant5 : Constant  Value=FS_LUT_TAU{7,1}.y  VectorParams1D=off
  Constant6 : Constant  Value=FS_LUT_TAU{7,1}.v  VectorParams1D=off
  Demux : Demux  Outputs=2
  MATLAB Function2 : MATLAB Function  TreatAsAtomicUnit=on
  Tau_bias : Outport
  wires:
  Constant5/1 -> MATLAB Function2/4(Y)
  Constant4/1 -> MATLAB Function2/3(X)
  [theta2] -> MATLAB Function2/1(theta)
  [delta2] -> MATLAB Function2/2(delta)
  MATLAB Function2/1(F) -> Tau_bias/1
  Constant6/1 -> MATLAB Function2/5(V)
  psi seg2/1 -> Demux/1
  Demux/1 -> [theta2]
  Demux/2 -> [delta2]

== system irep_force_control_m15/Wrench Estimation/tau sensing compensation/tau sensing compensation LUT/tau seg2 bias LUT/tau8_bias_neg ==
  psi seg2 : Inport
  Enable : EnablePort
  Constant1 : Constant  Value=FS_LUT_TAU{8,2}.x  VectorParams1D=off
  Constant2 : Constant  Value=FS_LUT_TAU{8,2}.y  VectorParams1D=off
  Constant3 : Constant  Value=FS_LUT_TAU{8,2}.v  VectorParams1D=off
  Demux : Demux  Outputs=2
  MATLAB Function1 : MATLAB Function  TreatAsAtomicUnit=on
  Tau_bias : Outport
  wires:
  MATLAB Function1/1(F) -> Tau_bias/1
  [delta2] -> MATLAB Function1/2(delta)
  [theta2] -> MATLAB Function1/1(theta)
  Constant2/1 -> MATLAB Function1/4(Y)
  Constant3/1 -> MATLAB Function1/5(V)
  Constant1/1 -> MATLAB Function1/3(X)
  psi seg2/1 -> Demux/1
  Demux/1 -> [theta2]
  Demux/2 -> [delta2]

== system irep_force_control_m15/Wrench Estimation/tau sensing compensation/tau sensing compensation LUT/tau seg2 bias LUT/tau8_bias_pos ==
  psi seg2 : Inport
  Enable : EnablePort
  Constant4 : Constant  Value=FS_LUT_TAU{8,1}.x  VectorParams1D=off
  Constant5 : Constant  Value=FS_LUT_TAU{8,1}.y  VectorParams1D=off
  Constant6 : Constant  Value=FS_LUT_TAU{8,1}.v  VectorParams1D=off
  Demux : Demux  Outputs=2
  MATLAB Function2 : MATLAB Function  TreatAsAtomicUnit=on
  Tau_bias : Outport
  wires:
  Constant6/1 -> MATLAB Function2/5(V)
  MATLAB Function2/1(F) -> Tau_bias/1
  [delta2] -> MATLAB Function2/2(delta)
  [theta2] -> MATLAB Function2/1(theta)
  Constant4/1 -> MATLAB Function2/3(X)
  Constant5/1 -> MATLAB Function2/4(Y)
  psi seg2/1 -> Demux/1
  Demux/1 -> [theta2]
  Demux/2 -> [delta2]

== system irep_force_control_m15/Trajectory Planner/Left Arm/High Level/Configuration Space/Parallelogram/5th Order Polynomial ==
  b des : Inport
  Digital Clock : DigitalClock  SampleTime=dt
  Embedded MATLAB Function : MATLAB Function  TreatAsAtomicUnit=on
  Unit Delay : UnitDelay  SampleTime=dt
  Unit Delay1 : UnitDelay  SampleTime=dt
  Unit Delay2 : UnitDelay  InitialCondition=[left_x0_parallelogram;z0_parallelogram]  SampleTime=dt
  tf : Constant  Value=5  SampleTime=dt
  b : Outport
  wires:
  tf/1 -> Embedded MATLAB Function/2(tf)
  Embedded MATLAB Function/1(pd) -> b/1
  b des/1 -> Embedded MATLAB Function/1(p_des)
  Digital Clock/1 -> Embedded MATLAB Function/3(tc)
  Unit Delay1/1 -> Embedded MATLAB Function/5(t0)
  Unit Delay2/1 -> Embedded MATLAB Function/6(p0)
  Embedded MATLAB Function/4(p0n) -> Unit Delay2/1
  Embedded MATLAB Function/3(t0n) -> Unit Delay1/1
  Unit Delay/1 -> Embedded MATLAB Function/4(conf)
  Embedded MATLAB Function/2(confn) -> Unit Delay/1

== system irep_force_control_m15/Trajectory Planner/Left Arm/High Level/Configuration Space/Stem/5th Order Polynomial ==
  psi des : Inport
  psi0 : Inport  Port=2
  enable : Inport  Port=3
  Digital Clock : DigitalClock  SampleTime=dt
  Embedded MATLAB Function : MATLAB Function  TreatAsAtomicUnit=on
  Unit Delay : UnitDelay  SampleTime=dt
  Unit Delay1 : UnitDelay  SampleTime=dt
  Unit Delay2 : UnitDelay  InitialCondition=zeros(5,1)  SampleTime=dt
  tf : Constant  Value=5  SampleTime=dt
  psi : Outport
  psi dot : Outport  Port=2
  wires:
  Embedded MATLAB Function/2(pdot) -> psi dot/1
  psi0/1 -> Embedded MATLAB Function/2(p_curr)
  enable/1 -> Embedded MATLAB Function/8(enable)
  tf/1 -> Embedded MATLAB Function/3(tf)
  Embedded MATLAB Function/1(p) -> psi/1
  psi des/1 -> Embedded MATLAB Function/1(p_des)
  Digital Clock/1 -> Embedded MATLAB Function/4(tc)
  Unit Delay1/1 -> Embedded MATLAB Function/6(t0)
  Unit Delay2/1 -> Embedded MATLAB Function/7(p0)
  Embedded MATLAB Function/5(p0n) -> Unit Delay2/1
  Embedded MATLAB Function/4(t0n) -> Unit Delay1/1
  Unit Delay/1 -> Embedded MATLAB Function/5(conf)
  Embedded MATLAB Function/3(confn) -> Unit Delay/1

== system irep_force_control_m15/Trajectory Planner/Right Arm/High Level/Configuration Space/Parallelogram/5th Order Polynomial ==
  b des : Inport
  Digital Clock : DigitalClock  SampleTime=dt
  Embedded MATLAB Function : MATLAB Function  TreatAsAtomicUnit=on
  Unit Delay : UnitDelay  SampleTime=dt
  Unit Delay1 : UnitDelay  SampleTime=dt
  Unit Delay2 : UnitDelay  InitialCondition=[x0_parallelogram;z0_parallelogram]  SampleTime=dt
  tf : Constant  Value=5  SampleTime=dt
  b : Outport
  wires:
  Embedded MATLAB Function/2(confn) -> Unit Delay/1
  Unit Delay/1 -> Embedded MATLAB Function/4(conf)
  Embedded MATLAB Function/3(t0n) -> Unit Delay1/1
  Embedded MATLAB Function/4(p0n) -> Unit Delay2/1
  Unit Delay2/1 -> Embedded MATLAB Function/6(p0)
  Unit Delay1/1 -> Embedded MATLAB Function/5(t0)
  Digital Clock/1 -> Embedded MATLAB Function/3(tc)
  b des/1 -> Embedded MATLAB Function/1(p_des)
  Embedded MATLAB Function/1(pd) -> b/1
  tf/1 -> Embedded MATLAB Function/2(tf)

== system irep_force_control_m15/Trajectory Planner/Right Arm/High Level/Configuration Space/Stem/5th Order Polynomial ==
  psi des : Inport
  psi0 : Inport  Port=2
  enable : Inport  Port=3
  Digital Clock : DigitalClock  SampleTime=dt
  Embedded MATLAB Function : MATLAB Function  TreatAsAtomicUnit=on
  Unit Delay : UnitDelay  SampleTime=dt
  Unit Delay1 : UnitDelay  SampleTime=dt
  Unit Delay2 : UnitDelay  InitialCondition=zeros(5,1)  SampleTime=dt
  tf : Constant  Value=5  SampleTime=dt
  psi : Outport
  psi dot : Outport  Port=2
  wires:
  Embedded MATLAB Function/3(confn) -> Unit Delay/1
  Unit Delay/1 -> Embedded MATLAB Function/5(conf)
  Embedded MATLAB Function/4(t0n) -> Unit Delay1/1
  Embedded MATLAB Function/5(p0n) -> Unit Delay2/1
  Unit Delay2/1 -> Embedded MATLAB Function/7(p0)
  Unit Delay1/1 -> Embedded MATLAB Function/6(t0)
  Digital Clock/1 -> Embedded MATLAB Function/4(tc)
  psi des/1 -> Embedded MATLAB Function/1(p_des)
  Embedded MATLAB Function/1(p) -> psi/1
  tf/1 -> Embedded MATLAB Function/3(tf)
  enable/1 -> Embedded MATLAB Function/8(enable)
  psi0/1 -> Embedded MATLAB Function/2(p_curr)
  Embedded MATLAB Function/2(pdot) -> psi dot/1

== matlab function irep_force_control_m15/Trajectory Planner/Right Arm/High Level/Inverse Istantaneous Kinematics/Coordination Module/Coordination Block ==
  data: b1 input; q1 output; q_par input; L0 input; q23 output
%--------------------------------------------------------------------------
%               Compute length of passive segment
%
%   Author: Andrea Bajo - andrea.bajo@vanderbilt.edu
%           Nabil Simaan - nabil.simaan@vanderbilt.edu
%
%           A.R.M.A. Lab
%           © 2010 Vanderbilt University
%
%   Created: 11:51 AM, October 22, 2010
%
%   Variables:
%       q1=q_ins+compensation insertion of the stem the passive stem.
%          q1=q_ins corresponds to straight stem configuration.
%       q_ins is the axial insertion of the passive stem (desired value).
%          q_ins=0 corresponds to the home position of the misumi slide.
%       q23 [q2;q3] is the desired postion of the parallelogram joints
%          with respect to straight configuration (right no b1 = [3.8;50.8])
%       b1=the desired position of the snake base=parallelogram tip in {B0}
%       {B0} is a right handed frame with z axis along center of IREP
%           stem and x axis pointing in the direction of parallelogram
%           opening
%       q_par=the corresponding q2, q3 values for the desired b1. 
%       L0=initial length of passive stem at home configuration. 
%       alpha is a compensation factor for accounting for the required pulling when the passive stem is commanded forward
%--------------------------------------------------------------------------
function [q1,q23]  = fcn(b1,q_par,L0)
%#eml

L = get_length_for_coordination(b1);
q_offset = L-L0;
q1 = q_offset;
q23 = q_par - [q_offset;q_offset];

== matlab function irep_force_control_m15/Trajectory Planner/Right Arm/High Level/Inverse Istantaneous Kinematics/5-Bar Inverse Kinematics ==
  data: b1 input; q output
function q  = fcn(b1)
%#eml
% if b1(1) > 3.8
%     x = b1(1)*1.6;
%     z = b1(2) - (b1(1)-3.8)/(20-3.8) * 6.5;
% else
    x = b1(1);
    z = b1(2);
% end
[q1 q2] = FiveBarInvKin(x,z);
q = [q1;q2];

== matlab function irep_force_control_m15/Trajectory Planner/RZ/Joystick Control for RZ/Embedded MATLAB Function ==
  data: u input; y output
function y = fcn(u)
%#eml

y = round(u*10)/10;

== matlab function irep_force_control_m15/Trajectory Planner/Right Arm/High Level/Task Space/Receive Desired Pose from MTM/Quaternion To Rotation ==
  data: quat input; R output
function R = fcn(quat)
%#eml
if norm(quat)==0
    quat = [1;0;0;0];
end
R = quat2rot(quat);

== matlab function irep_force_control_m15/Trajectory Planner/Right Arm/High Level/Configuration Space/Parallelogram/5th Order Polynomial/Embedded MATLAB Function ==
  data: p_des input; tf input; tc input; pd output; conf input; confn output; t0 input; t0n output; p0n output; p0 input
function [pd,confn,t0n,p0n] = fifth_order_p(p_des,tf,tc,conf,t0,p0)

% if enable == 0                  % Configuration space is not used (pdot = 0). 
%     p = p_curr;          % However we do want to record the current 
%     confn = 0;                  % position in order to be ready as soon 
%     t0n = tc;                   % as the enable becomes 1. 
%     p0n = p_curr;
% else
    if (p_des-p0)'*(p_des-p0) > 0
        if conf == 0                % conf = 0 means that the 5th order poly 
            p0n = p0;               % is not configured for the desired trajectory.
            t0n = tc;               % Therefore, the block is initialized.
            confn = 1;
            pd = zeros(2,1);
%              p = p0;
        else
            p0n = p0;
            t0n = t0;
            confn = conf;
            % 5th order polynomial
            a0 = p0;
            a4 = -15*(p_des-p0);
            a3 = -2/3 * a4;
            a5 = -2/5 * a4;
            t = tc-t0;
%             tau = t/tf;
            if t < tf
%                 p = a0 + a3 * tau^3 + a4 * tau^4 + a5 * tau^5;
                pd = 3*a3*t^2/tf^3 + 4*a4*t^3/tf^4 + 5*a5*t^4/tf^5;
            else
%                 p = p_des;
                pd = zeros(2,1);
                p0n = p_des;
            end
        end
    else
%         p = p_des;
        pd = zeros(2,1);
        confn = 0;
        p0n = p0;
        t0n = t0;
    end
% end
%------------------------------------------------------------------------

== matlab function irep_force_control_m15/Trajectory Planner/Right Arm/High Level/Inverse Istantaneous Kinematics/Coordination Module/5-Bar Inverse Kinematics ==
  data: b1 input; q output
function q  = fcn(b1)
%#eml
x = b1(1);
z = b1(2);
[q1 q2] = FiveBarInvKin(x,z);
q = [q1;q2];

== matlab function irep_force_control_m15/Trajectory Planner/Left Arm/High Level/Configuration Space/Parallelogram/5th Order Polynomial/Embedded MATLAB Function ==
  data: p_des input; tf input; tc input; pd output; conf input; confn output; t0 input; t0n output; p0n output; p0 input
function [pd,confn,t0n,p0n] = fifth_order_p(p_des,tf,tc,conf,t0,p0)

% if enable == 0                  % Configuration space is not used (pdot = 0). 
%     p = p_curr;          % However we do want to record the current 
%     confn = 0;                  % position in order to be ready as soon 
%     t0n = tc;                   % as the enable becomes 1. 
%     p0n = p_curr;
% else
    if (p_des-p0)'*(p_des-p0) > 0
        if conf == 0                % conf = 0 means that the 5th order poly 
            p0n = p0;               % is not configured for the desired trajectory.
            t0n = tc;               % Therefore, the block is initialized.
            confn = 1;
            pd = zeros(2,1);
%              p = p0;
        else
            p0n = p0;
            t0n = t0;
            confn = conf;
            % 5th order polynomial
            a0 = p0;
            a4 = -15*(p_des-p0);
            a3 = -2/3 * a4;
            a5 = -2/5 * a4;
            t = tc-t0;
%             tau = t/tf;
            if t < tf
%                 p = a0 + a3 * tau^3 + a4 * tau^4 + a5 * tau^5;
                pd = 3*a3*t^2/tf^3 + 4*a4*t^3/tf^4 + 5*a5*t^4/tf^5;
            else
%                 p = p_des;
                pd = zeros(2,1);
                p0n = p_des;
            end
        end
    else
%         p = p_des;
        pd = zeros(2,1);
        confn = 0;
        p0n = p0;
        t0n = t0;
    end
% end
%------------------------------------------------------------------------

== matlab function irep_force_control_m15/Trajectory Planner/Left Arm/High Level/Configuration Space/Stem/5th Order Polynomial/Embedded MATLAB Function ==
  data: p_des input; p_curr input; tf input; tc input; p output; pdot output; conf input; confn output; t0 input; t0n output; p0n output; p0 input; enable input
function [p,pdot,confn,t0n,p0n] = fifth_order_p(p_des,p_curr,tf,tc,conf,t0,p0,enable)

if enable == 0                  % Configuration space is not used (pdot = 0). 
    p = p_curr;          % However we do want to record the current 
    confn = 0;                  % position in order to be ready as soon 
    t0n = tc;                   % as the enable becomes 1. 
    p0n = p_curr;
    pdot = zeros(5,1);
else
    if (p_des-p0)'*(p_des-p0) > 0
        if conf == 0                % conf = 0 means that the 5th order poly 
            p0n = p0;               % is not configured for the desired trajectory.
            t0n = tc;               % Therefore, the block is initialized.
            confn = 1;
            p = p0;
            pdot = zeros(5,1);
        else
            p0n = p0;
            t0n = t0;
            confn = conf;
            % 5th order polynomial
            a0 = p0;
            a4 = -15*(p_des-p0);
            a3 = -2/3 * a4;
            a5 = -2/5 * a4;
            t = tc-t0;
            tau = t/tf;
            if t < tf
                p = a0 + a3 * tau^3 + a4 * tau^4 + a5 * tau^5;
                pdot = 3*a3*t^2/tf^3 + 4*a4*t^3/tf^4 + 5*a5*t^4/tf^5;
            else
                p = p_des;
                pdot = zeros(5,1);
                p0n = p_des;
            end
        end
    else
        p = p_des;
        pdot = zeros(5,1);
        confn = 0;
        p0n = p0;
        t0n = t0;
    end
end
%------------------------------------------------------------------------

== matlab function irep_force_control_m15/Trajectory Planner/Camera/Homing Procedure/Homing Completion ==
  data: u input; y output
function y = fcn(u)
%#codegen
y = zeros(3,1);
u = abs(u);
if u(1) <= 0.002
    y(1) = 1;
end
if u(2) <= 0.002
    y(2) = 1;
end
if u(3) <= 0.002
    y(3) = 1;
end

== matlab function irep_force_control_m15/Trajectory Planner/Left Arm/High Level/Inverse Istantaneous Kinematics/5-Bar Inverse Kinematics ==
  data: b1 input; q output
function q  = fcn(b1)
%#eml
b1 = [-b1(1);b1(2)];

x = b1(1);
z = b1(2);

[q1 q2] = FiveBarInvKin(x,z);
q = [q1;q2];

== matlab function irep_force_control_m15/Trajectory Planner/Left Arm/High Level/Inverse Istantaneous Kinematics/Coordination Module/5-Bar Inverse Kinematics ==
  data: b1 input; q output
function q  = fcn(b1)
%#eml
x = b1(1);
z = b1(2);
[q1 q2] = FiveBarInvKin(x,z);
q = [q1;q2];

== matlab function irep_force_control_m15/Trajectory Planner/Left Arm/High Level/Inverse Istantaneous Kinematics/Coordination Module/Coordination Block ==
  data: b1 input; q1 output; q_par input; L0 input; q23 output
%--------------------------------------------------------------------------
%               Compute length of passive segment
%
%   Author: Andrea Bajo - andrea.bajo@vanderbilt.edu
%           Nabil Simaan - nabil.simaan@vanderbilt.edu
%
%           A.R.M.A. Lab
%           © 2010 Vanderbilt University
%
%   Created: 11:51 AM, October 22, 2010
%
%   Variables:
%       q1=q_ins+compensation insertion of the stem the passive stem.
%          q1=q_ins corresponds to straight stem configuration.
%       q_ins is the axial insertion of the passive stem (desired value).
%          q_ins=0 corresponds to the home position of the misumi slide.
%       q23 [q2;q3] is the desired postion of the parallelogram joints
%          with respect to straight configuration (right no b1 = [3.8;50.8])
%       b1=the desired position of the snake base=parallelogram tip in {B0}
%       {B0} is a right handed frame with z axis along center of IREP
%           stem and x axis pointing in the direction of parallelogram
%           opening
%       q_par=the corresponding q2, q3 values for the desired b1. 
%       L0=initial length of passive stem at home configuration. 
%       alpha is a compensation factor for accounting for the required pulling when the passive stem is commanded forward
%--------------------------------------------------------------------------
function [q1,q23]  = fcn(b1,q_par,L0)
%#eml
L = get_length_for_coordination([-b1(1);b1(2)]);
q_offset = L-L0;
% q1 = beta*q_offset; %insertion axis
q1 = q_offset; %insertion axis
% q23 = q_par - alpha*[q_offset;q_offset];
q23 = q_par - [q_offset;q_offset];
